simulink model "Imitation_Task_Multi_withSound_withGrid"  (R2015a)
settings: Solver=ode4  SolverMode=MultiTasking  StartTime=0.0  StopTime=inf  FixedStep=BKIN_STEP_TIME  RelTol=1e-3
StartFcn:
  |  warndlg('Dexterit-E models cannot run under simulation. Please compile your model and run it from within Dexterit-E.');set_param(bdroot,'SimulationCommand','stop')
model workspace (MAT data in the model file):
  col_x = 1
  col_y = 2
  RADIUS_VIS = 3
  COLOR_INIT = 4
  START_TARGET_COL = 1
  DELAY_POST_TRIAL_COL = 20
  BKIN_STEP_TIME = 0.00025
  COLOR_MOVE = 5
  START_WAIT_TIME_COL = 2
  CUE_TARGET_COL = 3
  STIM_DUR_COL = 17
  MAX_MOVE_TIME_COL = 18
  HOLD_TIME_COL = 19
  E_START_TRIAL = 2
  E_START_REACHED = 4
  E_MOVED_EARLY = 21
  E_GO_CUE = 9
  E_MOVE_TIMEOUT = 23
  E_HOLDING_STILL = 12
  E_END_TRIAL = 14
  CONTROL_PT1_COL = 8
  CONTROL_PT2_COL = 9
  CONTROL_PT3_COL = 10
  CONTROL_PT4_COL = 11
  STROKE_WIDTH = 6
  K_HAND_VEL = 1
  E_MOVE_ON = 10
  CUE_TYPE_COL = 6
  CUE_VIS_COL = 4
  HAND_VIS_COL = 5
  K_HOLDTIME = 2
  K_ROBOT_RAMP_TIME = 3
  E_ROBOT_RETURN_TO_START = 33
  E_ENABLED_CONTROLLER = 31
  K_TIME_TO_START = 4
  E_RETURN_TO_START = 35
  E_HOLD_POS = 37
  CONTROL_PT5_COL = 12
  CONTROL_PT6_COL = 13
  CONTROL_PT7_COL = 14
  CONTROL_PT8_COL = 15
  CONTROL_PT9_COL = 16
  E_INCREMENTING_TSTEP1 = 6
  E_INCREMENTING_TSTEP2 = 7
  E_INCREMENTING_TSTEP3 = 8
  CONTROL_PT0_COL = 7
  K_TONE_START_FREQUENCY = 5
  K_TONE_START_DURATION = 6
  K_TONE_GO_FREQUENCY = 7
  K_TONE_GO_DURATION = 8
  ENABLE_BKGND_GRID_COL = 21
  BKGND_GRID_TGT_COL = 22
  BKIN_KINEMATIC_FRAME_SIZE = 400
  E_NO_EVENT = 0
  END_REACH_BUTTON = 2
  E_BUTTON_ON = 40
libraries: slrtlib x9, Video x7, General x3, KINARM_general x2, KINARM_loads x2, simulink x1, xpcnilib x1
(part 2 of 2)

== matlab function Imitation_Task_Multi_withSound_withGrid/Subsystem1/MATLAB Function ==
  data: VCODE input; VCODES_GRID output size=[25 70]; StartTgtVCODE input
function VCODES_GRID  = fcn(VCODE,StartTgtVCODE)
%#codegen

%we will tile the space between (+x/-x, +y/0) at regular intervals

xmax = VCODE(3);
ymax = VCODE(4);

%xs = linspace(-xmax,xmax,Nx);
%ys = linspace(0,ymax,Ny);
xs = zeros(5,1);  %we will set the grid to always be 5 by 5 since Simulink doesn't like variable-lenth variables
ys = zeros(5,1);

startX = StartTgtVCODE(3);
startY = StartTgtVCODE(4);

xmax = abs(xmax-startX);  %get the offset relative to the start target
ymax = abs(ymax-startY);

for a = 1:5

    
    xs(a) = -xmax + (xmax*2)/4*(a-1);
    ys(a) = 0 + (ymax)/4*(a-1);
end

[gridX,gridY] = meshgrid(xs,ys);
grid = [reshape(gridX,[],1),reshape(gridY,[],1)];

%VCODE(1) = VCODE(1)+ 100;  %mark as a background target

%we will initialize this to be 30; we won't allow any more points than
%this!
VCODES_GRID = zeros(25,70);

%VCODES_GRID = repmat(VCODE,size(grid,1),1);

for a = 1:min(size(grid,1),25)
    VCODES_GRID(a,:) = VCODE;
    VCODES_GRID(a,3) = grid(a,1)+startX;
    VCODES_GRID(a,4) = grid(a,2)+startY;
    VCODES_GRID(a,8) = a+50;  %set the ID
end

pos = VCODES_GRID(:,3:4);
gridpos = reshape(pos',[],1);

== matlab function Imitation_Task_Multi_withSound_withGrid/Play Sound/Play sound over and over ==
  data: tone input; output output; beep input; beep1 input; beep2 input
function output = fcn(tone,beep,beep1,beep2)
%#codegen

persistent t last_tone_state
if isempty(t), t = 0; end
if isempty(last_tone_state), last_tone_state = 0; end

trigger = last_tone_state ~= tone;
if trigger > 0
    last_tone_state = tone;
end

output = 0;		% default
if t == 0 && trigger > 0
	% start the playing of the sound.
	t = t + 1;
end

if tone == 1
    data = beep;
elseif tone == 2
    data = beep1;
elseif tone == 3
    data = beep2;
else 
    t = 0;
    data = 0;
end

if t > 0
	output = data(t);
	if t == length(data)
		t = 0;
	else
		t = t + 1;
	end
end
